simulink model "Automated_BCM_Integrated_2020b"  (R2020b)
settings: Solver=VariableStepAuto  StartTime=0.0  StopTime=100  RelTol=1e-3
undefined symbols (not defined in the file): sigbuilder_block
settings Model: EnablePacing=on  PacingRate=2  Creator=99003729  LastModifiedBy=99003729

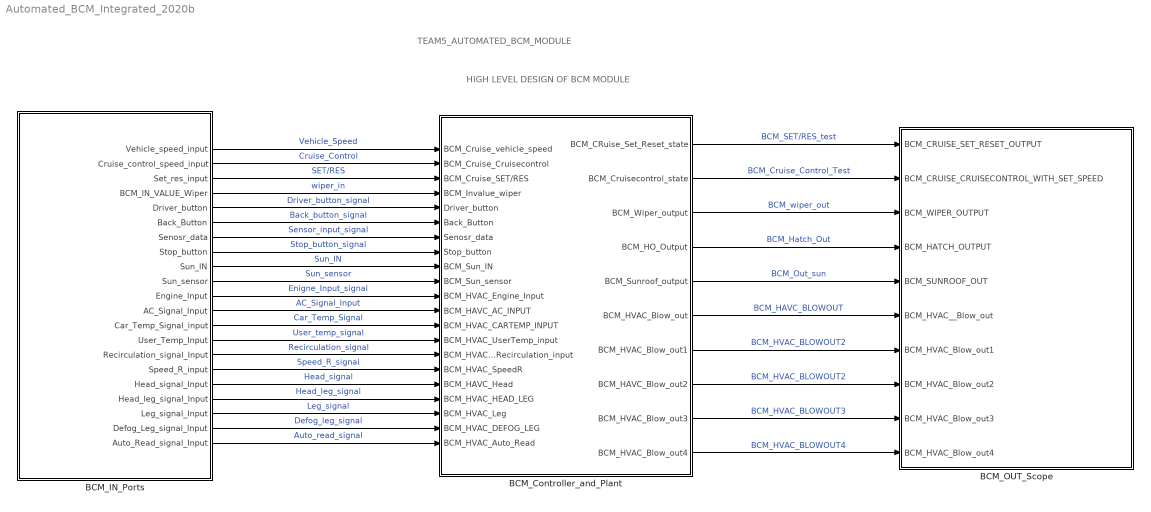
== system Automated_BCM_Integrated_2020b ==
  note: HIGH LEVEL DESIGN OF BCM MODULE
  note: TEAM5_AUTOMATED_BCM_MODULE
  BCM_Controller_and_Plant : Subsystem
  BCM_IN_Ports : Subsystem
  BCM_OUT_Scope : Subsystem
  wires:
  BCM_IN_Ports/1(Vehicle_speed_input) -> BCM_Controller_and_Plant/1(BCM_Cruise_vehicle_speed)  "Vehicle_Speed"
  BCM_IN_Ports/3(Set_res_input) -> BCM_Controller_and_Plant/3(BCM_Cruise_SET/RES)  "SET/RES"
  BCM_IN_Ports/2(Cruise_control_speed_input) -> BCM_Controller_and_Plant/2(BCM_Cruise_Cruisecontrol)  "Cruise_Control"
  BCM_Controller_and_Plant/1(BCM_CRuise_Set_Reset_state) -> BCM_OUT_Scope/1(BCM_CRUISE_SET_RESET_OUTPUT)  "BCM_SET/RES_test"
  BCM_Controller_and_Plant/2(BCM_Cruisecontrol_state) -> BCM_OUT_Scope/2(BCM_CRUISE_CRUISECONTROL_WITH_SET_SPEED)  "BCM_Cruise_Control_Test"
  BCM_IN_Ports/4(BCM_IN_VALUE_Wiper) -> BCM_Controller_and_Plant/4(BCM_Invalue_wiper)  "wiper_in"
  BCM_Controller_and_Plant/3(BCM_Wiper_output) -> BCM_OUT_Scope/3(BCM_WIPER_OUTPUT)  "BCM_wiper_out"
  BCM_Controller_and_Plant/4(BCM_HO_Output) -> BCM_OUT_Scope/4(BCM_HATCH_OUTPUT)  "BCM_Hatch_Out"
  BCM_IN_Ports/5(Driver_button) -> BCM_Controller_and_Plant/5(Driver_button)  "Driver_button_signal"
  BCM_IN_Ports/6(Back_Button) -> BCM_Controller_and_Plant/6(Back_Button)  "Back_button_signal"
  BCM_IN_Ports/7(Senosr_data) -> BCM_Controller_and_Plant/7(Senosr_data)  "Sensor_input_signal"
  BCM_IN_Ports/8(Stop_button) -> BCM_Controller_and_Plant/8(Stop_button)  "Stop_button_signal"
  BCM_Controller_and_Plant/5(BCM_Sunroof_output) -> BCM_OUT_Scope/5(BCM_SUNROOF_OUT)  "BCM_Out_sun"
  BCM_IN_Ports/9(Sun_IN) -> BCM_Controller_and_Plant/9(BCM_Sun_IN)  "Sun_IN"
  BCM_IN_Ports/10(Sun_sensor) -> BCM_Controller_and_Plant/10(BCM_Sun_sensor)  "Sun_sensor"
  BCM_IN_Ports/11(Engine_Input) -> BCM_Controller_and_Plant/11(BCM_HVAC_Engine_Input)  "Enigne_Input_signal"
  BCM_IN_Ports/12(AC_Signal_Input) -> BCM_Controller_and_Plant/12(BCM_HAVC_AC_INPUT)  "AC_Signal_Input"
  BCM_IN_Ports/13(Car_Temp_Signal_input) -> BCM_Controller_and_Plant/13(BCM_HVAC_CARTEMP_INPUT)  "Car_Temp_Signal"
  BCM_IN_Ports/14(User_Temp_Input) -> BCM_Controller_and_Plant/14(BCM_HVAC_UserTemp_input)  "User_temp_signal"
  BCM_IN_Ports/15(Recirculation_signal_Input) -> BCM_Controller_and_Plant/15(BCM_HVAC_Recirculation_input)  "Recirculation_signal"
  BCM_IN_Ports/16(Speed_R_input) -> BCM_Controller_and_Plant/16(BCM_HVAC_SpeedR)  "Speed_R_signal"
  BCM_IN_Ports/17(Head_signal_Input) -> BCM_Controller_and_Plant/17(BCM_HAVC_Head)  "Head_signal"
  BCM_IN_Ports/18(Head_leg_signal_Input) -> BCM_Controller_and_Plant/18(BCM_HVAC_HEAD_LEG)  "Head_leg_signal"
  BCM_IN_Ports/19(Leg_signal_Input) -> BCM_Controller_and_Plant/19(BCM_HVAC_Leg)  "Leg_signal"
  BCM_IN_Ports/20(Defog_Leg_signal_Input) -> BCM_Controller_and_Plant/20(BCM_HVAC_DEFOG_LEG)  "Defog_leg_signal"
  BCM_IN_Ports/21(Auto_Read_signal_Input) -> BCM_Controller_and_Plant/21(BCM_HVAC_Auto_Read)  "Auto_read_signal"
  BCM_Controller_and_Plant/6(BCM_HVAC_Blow_out) -> BCM_OUT_Scope/6(BCM_HVAC__Blow_out)  "BCM_HAVC_BLOWOUT"
  BCM_Controller_and_Plant/7(BCM_HVAC_Blow_out1) -> BCM_OUT_Scope/7(BCM_HVAC_Blow_out1)  "BCM_HVAC_BLOWOUT2"
  BCM_Controller_and_Plant/8(BCM_HAVC_Blow_out2) -> BCM_OUT_Scope/8(BCM_HVAC_Blow_out2)  "BCM_HVAC_BLOWOUT2"
  BCM_Controller_and_Plant/9(BCM_HVAC_Blow_out3) -> BCM_OUT_Scope/9(BCM_HVAC_Blow_out3)  "BCM_HVAC_BLOWOUT3"
  BCM_Controller_and_Plant/10(BCM_HVAC_Blow_out4) -> BCM_OUT_Scope/10(BCM_HVAC_Blow_out4)  "BCM_HVAC_BLOWOUT4"

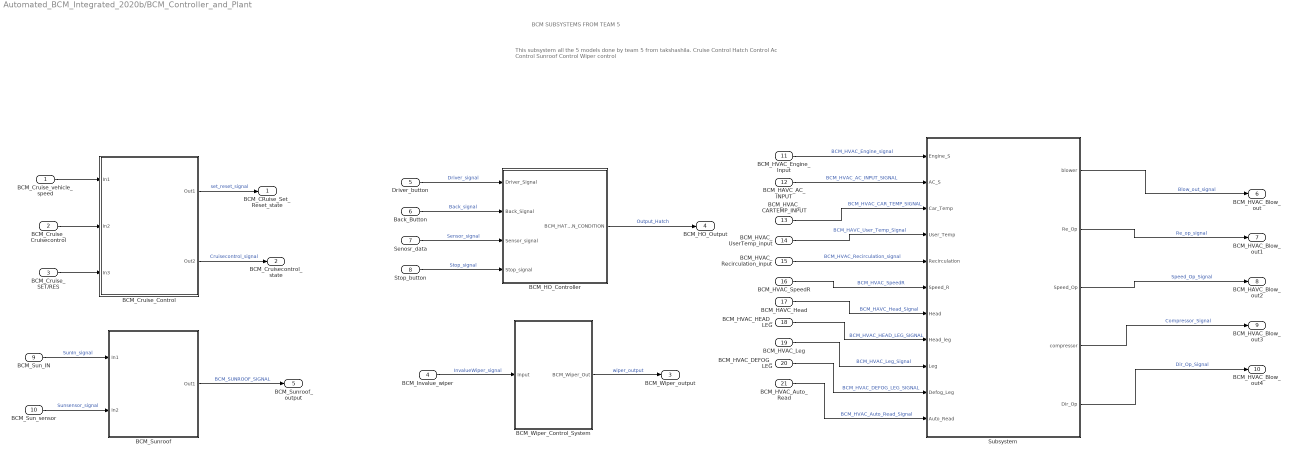
== system Automated_BCM_Integrated_2020b/BCM_Controller_and_Plant ==
  note: This subsystem all the 5 models done by team 5 from takshashila.
      | Cruise Control
      | Hatch Control
      | Ac Control
      | Sunroof Control
      | Wiper control
  note: BCM SUBSYSTEMS FROM TEAM 5
  BCM_Cruise_vehicle_speed : Inport
  BCM_Cruise_Cruisecontrol : Inport  Port=2
  BCM_Cruise_SET/RES : Inport  Port=3
  BCM_Invalue_wiper : Inport  Port=4
  Driver_button : Inport  Port=5
  Back_Button : Inport  Port=6
  Senosr_data : Inport  Port=7
  Stop_button : Inport  Port=8
  BCM_Sun_IN : Inport  Port=9
  BCM_Sun_sensor : Inport  Port=10
  BCM_HVAC_Engine_Input : Inport  Port=11
  BCM_HAVC_AC_INPUT : Inport  Port=12
  BCM_HVAC_CARTEMP_INPUT : Inport  Port=13
  BCM_HVAC_UserTemp_input : Inport  Port=14
  BCM_HVAC_Recirculation_input : Inport  Port=15
  BCM_HVAC_SpeedR : Inport  Port=16
  BCM_HAVC_Head : Inport  Port=17
  BCM_HVAC_HEAD_LEG : Inport  Port=18
  BCM_HVAC_Leg : Inport  Port=19
  BCM_HVAC_DEFOG_LEG : Inport  Port=20
  BCM_HVAC_Auto_Read : Inport  Port=21
  BCM_Cruise_Control : Subsystem
  BCM_HO_Controller : Subsystem
  BCM_Sunroof : Subsystem
  BCM_Wiper_Control_System : Subsystem
  Subsystem : Subsystem
  BCM_CRuise_Set_Reset_state : Outport
  BCM_Cruisecontrol_state : Outport  Port=2
  BCM_Wiper_output : Outport  Port=3
  BCM_HO_Output : Outport  Port=4
  BCM_Sunroof_output : Outport  Port=5
  BCM_HVAC_Blow_out : Outport  Port=6
  BCM_HVAC_Blow_out1 : Outport  Port=7
  BCM_HAVC_Blow_out2 : Outport  Port=8
  BCM_HVAC_Blow_out3 : Outport  Port=9
  BCM_HVAC_Blow_out4 : Outport  Port=10
  wires:
  BCM_Cruise_vehicle_speed/1 -> BCM_Cruise_Control/1(In1)
  BCM_Cruise_Cruisecontrol/1 -> BCM_Cruise_Control/2(In2)
  BCM_Cruise_SET/RES/1 -> BCM_Cruise_Control/3(In3)
  BCM_Cruise_Control/1(Out1) -> BCM_CRuise_Set_Reset_state/1  "set_reset_signal"
  BCM_Cruise_Control/2(Out2) -> BCM_Cruisecontrol_state/1  "Cruisecontrol_signal"
  Driver_button/1 -> BCM_HO_Controller/1(Driver_Signal)  "Driver_signal"
  Back_Button/1 -> BCM_HO_Controller/2(Back_Signal)  "Back_signal"
  Senosr_data/1 -> BCM_HO_Controller/3(Sensor_signal)  "Sensor_signal"
  Stop_button/1 -> BCM_HO_Controller/4(Stop_signal)  "Stop_signal"
  BCM_Sunroof/1(Out1) -> BCM_Sunroof_output/1  "BCM_SUNROOF_SIGNAL"
  BCM_Sun_IN/1 -> BCM_Sunroof/1(In1)  "SunIn_signal"
  BCM_Sun_sensor/1 -> BCM_Sunroof/2(In2)  "Sunsensor_signal"
  BCM_Invalue_wiper/1 -> BCM_Wiper_Control_System/1(Input)  "InvalueWiper_signal"
  BCM_Wiper_Control_System/1(BCM_Wiper_Out) -> BCM_Wiper_output/1  "wiper_output"
  BCM_HO_Controller/1(BCM_HATCHOPEN_CONDITION) -> BCM_HO_Output/1  "Output_Hatch"
  BCM_HVAC_Engine_Input/1 -> Subsystem/1(Engine_S)  "BCM_HVAC_Engine_signal"
  BCM_HAVC_AC_INPUT/1 -> Subsystem/2(AC_S)  "BCM_HVAC_AC_INPUT_SIGNAL"
  BCM_HVAC_CARTEMP_INPUT/1 -> Subsystem/3(Car_Temp)  "BCM_HVAC_CAR_TEMP_SIGNAL"
  BCM_HVAC_UserTemp_input/1 -> Subsystem/4(User_Temp)  "BCM_HAVC_User_Temp_Signal"
  BCM_HVAC_Recirculation_input/1 -> Subsystem/5(Recirculation)  "BCM_HVAC_Recirculation_signal"
  BCM_HVAC_SpeedR/1 -> Subsystem/6(Speed_R)  "BCM_HVAC_SpeedR"
  BCM_HAVC_Head/1 -> Subsystem/7(Head)  "BCM_HAVC_Head_Signal"
  BCM_HVAC_HEAD_LEG/1 -> Subsystem/8(Head_leg)  "BCM_HVAC_HEAD_LEG_SIGNAL"
  BCM_HVAC_Leg/1 -> Subsystem/9(Leg)  "BCM_HVAC_Leg_Signal"
  BCM_HVAC_DEFOG_LEG/1 -> Subsystem/10(Defog_Leg)  "BCM_HVAC_DEFOG_LEG_SIGNAL"
  BCM_HVAC_Auto_Read/1 -> Subsystem/11(Auto_Read)  "BCM_HVAC_Auto_Read_Signal"
  Subsystem/1(blower) -> BCM_HVAC_Blow_out/1  "Blow_out_signal"
  Subsystem/2(Re_Op) -> BCM_HVAC_Blow_out1/1  "Re_op_signal"
  Subsystem/3(Speed_Op) -> BCM_HAVC_Blow_out2/1  "Speed_Op_Signal"
  Subsystem/4(compressor) -> BCM_HVAC_Blow_out3/1  "Compressor_Signal"
  Subsystem/5(Dir_Op) -> BCM_HVAC_Blow_out4/1  "Dir_Op_Signal"

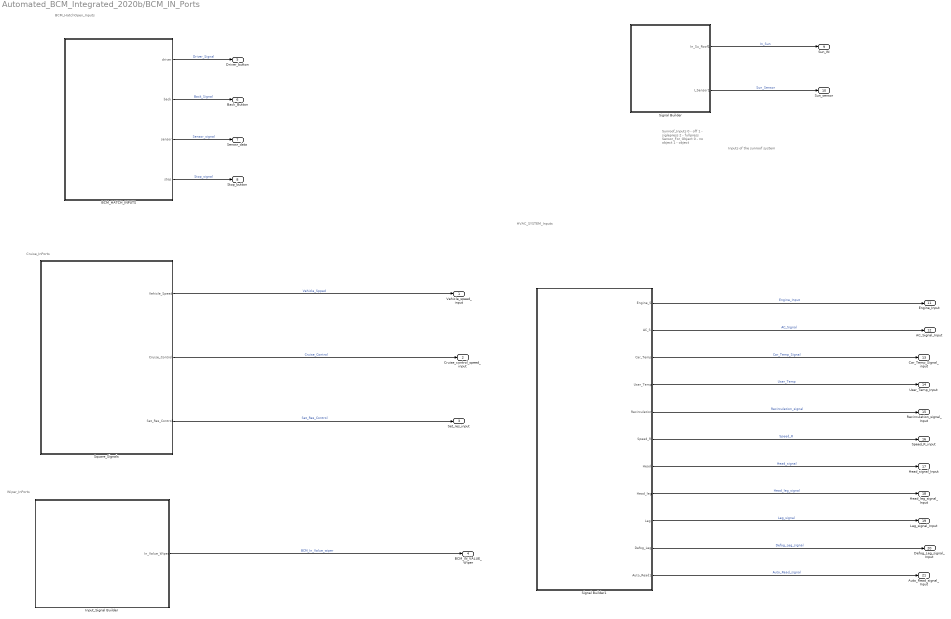
== system Automated_BCM_Integrated_2020b/BCM_IN_Ports ==
  note: HVAC_SYSTEM_Inputs
  note: BCM_HatchOpen_Inputs
  note: Wiper_InPorts
  note: Cruise_InPorts
  note: Inputs of the sunroof system
  note: Sunroof_Inputs
      | 0 - off
      | 1 - siglepress
      | 2 - fullpress
      | Sensor_For_Object
      | 0 - no object
      | 1 - object
  BCM_HATCH_INPUTS : Subsystem  Tag=STV Subsys  LoadFcn=sigbuilder_block('load');  StartFcn=sigbuilder_block('start');  StopFcn=sigbuilder_block('stop');  ClipboardFcn=sigbuilder_block('clipboard');  mask(Sigbuilder block){tuvar=[0:10]}
      mask help: Simulink:masks:SigbuilderBlock_MD
      mask init:
      | if ~strcmp(get_param(bdroot(gcbh),'SimulationStatus'),'stopped') tuvar = sigbuilder_block('maskInit'); end
      settings: CopyFcn=sigbuilder_block('copy');  DeleteFcn=sigbuilder_block('delete');  ModelCloseFcn=sigbuilder_block('modelClose');  PreSaveFcn=sigbuilder_block('preSave');  PauseFcn=sigbuilder_block('pause');  ContinueFcn=sigbuilder_block('continue');  NameChangeFcn=sigbuilder_block('namechange');  OpenFcn=sigbuilder_block('open',[0 30 1440 722.25 ]);  CloseFcn=sigbuilder_block('close');
      mask Display: plot(0, 0, 100, 100,[2, 2, 32, 32, 2], [68, 8, 8, 68, 68],[32, 2], [38, 38], [32, 19, 2],[53, 60, 44], [32, 17, 17, 2],[16, 16, 31, 31]);txt = getActiveGroup(gcbh);text(2, 100, txt,'verticalAlignment', 'top');
  Input_Signal Builder : Subsystem  Tag=STV Subsys  LoadFcn=sigbuilder_block('load');  StartFcn=sigbuilder_block('start');  StopFcn=sigbuilder_block('stop');  ClipboardFcn=sigbuilder_block('clipboard');  mask(Sigbuilder block){tuvar=[0:10]}
      mask help: Simulink:masks:SigbuilderBlock_MD
      mask init:
      | if ~strcmp(get_param(bdroot(gcbh),'SimulationStatus'),'stopped') tuvar = sigbuilder_block('maskInit'); end
      settings: CopyFcn=sigbuilder_block('copy');  DeleteFcn=sigbuilder_block('delete');  ModelCloseFcn=sigbuilder_block('modelClose');  PreSaveFcn=sigbuilder_block('preSave');  PauseFcn=sigbuilder_block('pause');  ContinueFcn=sigbuilder_block('continue');  NameChangeFcn=sigbuilder_block('namechange');  OpenFcn=sigbuilder_block('open',[339 188.25 550.5 359.25 ]);  CloseFcn=sigbuilder_block('close');
      mask Display: plot(0, 0, 100, 100,[2, 2, 32, 32, 2], [68, 8, 8, 68, 68],[32, 2], [38, 38], [32, 19, 2],[53, 60, 44], [32, 17, 17, 2],[16, 16, 31, 31]);txt = getActiveGroup(gcbh);text(2, 100, txt,'verticalAlignment', 'top');
  Signal Builder : Subsystem  Tag=STV Subsys  LoadFcn=sigbuilder_block('load');  StartFcn=sigbuilder_block('start');  StopFcn=sigbuilder_block('stop');  ClipboardFcn=sigbuilder_block('clipboard');  mask(Sigbuilder block){tuvar=[0:10]}
      mask help: Simulink:masks:SigbuilderBlock_MD
      mask init:
      | if ~strcmp(get_param(bdroot(gcbh),'SimulationStatus'),'stopped') tuvar = sigbuilder_block('maskInit'); end
      settings: CopyFcn=sigbuilder_block('copy');  DeleteFcn=sigbuilder_block('delete');  ModelCloseFcn=sigbuilder_block('modelClose');  PreSaveFcn=sigbuilder_block('preSave');  PauseFcn=sigbuilder_block('pause');  ContinueFcn=sigbuilder_block('continue');  NameChangeFcn=sigbuilder_block('namechange');  OpenFcn=sigbuilder_block('open',[534 -108 550.5 359.25 ]);  CloseFcn=sigbuilder_block('close');
      mask Display: plot(0, 0, 100, 100,[2, 2, 32, 32, 2], [68, 8, 8, 68, 68],[32, 2], [38, 38], [32, 19, 2],[53, 60, 44], [32, 17, 17, 2],[16, 16, 31, 31]);txt = getActiveGroup(gcbh);text(2, 100, txt,'verticalAlignment', 'top');
  Signal Builder1 : Subsystem  Tag=STV Subsys  LoadFcn=sigbuilder_block('load');  StartFcn=sigbuilder_block('start');  StopFcn=sigbuilder_block('stop');  ClipboardFcn=sigbuilder_block('clipboard');  mask(Sigbuilder block){tuvar=[0:10]}
      mask help: Simulink:masks:SigbuilderBlock_MD
      mask init:
      | if ~strcmp(get_param(bdroot(gcbh),'SimulationStatus'),'stopped') tuvar = sigbuilder_block('maskInit'); end
      settings: CopyFcn=sigbuilder_block('copy');  DeleteFcn=sigbuilder_block('delete');  ModelCloseFcn=sigbuilder_block('modelClose');  PreSaveFcn=sigbuilder_block('preSave');  PauseFcn=sigbuilder_block('pause');  ContinueFcn=sigbuilder_block('continue');  NameChangeFcn=sigbuilder_block('namechange');  OpenFcn=sigbuilder_block('open',[417 237.75 550.5 399.75 ]);  CloseFcn=sigbuilder_block('close');
      mask Display: plot(0, 0, 100, 100,[2, 2, 32, 32, 2], [68, 8, 8, 68, 68],[32, 2], [38, 38], [32, 19, 2],[53, 60, 44], [32, 17, 17, 2],[16, 16, 31, 31]);txt = getActiveGroup(gcbh);text(2, 100, txt,'verticalAlignment', 'top');
  Square_Signals : Subsystem  Tag=STV Subsys  LoadFcn=sigbuilder_block('load');  StartFcn=sigbuilder_block('start');  StopFcn=sigbuilder_block('stop');  ClipboardFcn=sigbuilder_block('clipboard');  mask(Sigbuilder block){tuvar=[0:10]}
      mask help: Simulink:masks:SigbuilderBlock_MD
      mask init:
      | if ~strcmp(get_param(bdroot(gcbh),'SimulationStatus'),'stopped') tuvar = sigbuilder_block('maskInit'); end
      settings: CopyFcn=sigbuilder_block('copy');  DeleteFcn=sigbuilder_block('delete');  ModelCloseFcn=sigbuilder_block('modelClose');  PreSaveFcn=sigbuilder_block('preSave');  PauseFcn=sigbuilder_block('pause');  ContinueFcn=sigbuilder_block('continue');  NameChangeFcn=sigbuilder_block('namechange');  OpenFcn=sigbuilder_block('open',[0.75 30.75 718.5 715.5 ]);  CloseFcn=sigbuilder_block('close');
      mask Display: plot(0, 0, 100, 100,[2, 2, 32, 32, 2], [68, 8, 8, 68, 68],[32, 2], [38, 38], [32, 19, 2],[53, 60, 44], [32, 17, 17, 2],[16, 16, 31, 31]);txt = getActiveGroup(gcbh);text(2, 100, txt,'verticalAlignment', 'top');
  Vehicle_speed_input : Outport
  Cruise_control_speed_input : Outport  Port=2
  Set_res_input : Outport  Port=3
  BCM_IN_VALUE_Wiper : Outport  Port=4
  Driver_button : Outport  Port=5
  Back_Button : Outport  Port=6
  Senosr_data : Outport  Port=7
  Stop_button : Outport  Port=8
  Sun_IN : Outport  Port=9
  Sun_sensor : Outport  Port=10
  Engine_Input : Outport  Port=11
  AC_Signal_Input : Outport  Port=12
  Car_Temp_Signal_input : Outport  Port=13
  User_Temp_Input : Outport  Port=14
  Recirculation_signal_Input : Outport  Port=15
  Speed_R_input : Outport  Port=16
  Head_signal_Input : Outport  Port=17
  Head_leg_signal_Input : Outport  Port=18
  Leg_signal_Input : Outport  Port=19
  Defog_Leg_signal_Input : Outport  Port=20
  Auto_Read_signal_Input : Outport  Port=21
  wires:
  Square_Signals/2(Cruise_Control) -> Cruise_control_speed_input/1  "Cruise_Control"
  Square_Signals/1(Vehicle_Speed) -> Vehicle_speed_input/1  "Vehicle_Spped"
  Square_Signals/3(Set_Res_Control) -> Set_res_input/1  "Set_Res_Control"
  Input_Signal Builder/1(In_Value_Wiper) -> BCM_IN_VALUE_Wiper/1  "BCM_In_Value_wiper"
  BCM_HATCH_INPUTS/4(stop) -> Stop_button/1  "Stop_signal"
  BCM_HATCH_INPUTS/3(sensor) -> Senosr_data/1  "Sensor_signal"
  BCM_HATCH_INPUTS/2(back) -> Back_Button/1  "Back_Signal"
  BCM_HATCH_INPUTS/1(driver) -> Driver_button/1  "Driver_Signal"
  Signal Builder/1(In_Su_Roof1) -> Sun_IN/1  "In_Sun"
  Signal Builder/2(I_Sensor1) -> Sun_sensor/1  "Sun_Sensor"
  Signal Builder1/8(Head_leg) -> Head_leg_signal_Input/1  "Head_leg_signal"
  Signal Builder1/9(Leg) -> Leg_signal_Input/1  "Leg_signal"
  Signal Builder1/4(User_Temp) -> User_Temp_Input/1  "User_Temp"
  Signal Builder1/6(Speed_R) -> Speed_R_input/1  "Speed_R"
  Signal Builder1/7(Head) -> Head_signal_Input/1  "Head_signal"
  Signal Builder1/3(Car_Temp) -> Car_Temp_Signal_input/1  "Car_Temp_Signal"
  Signal Builder1/10(Defog_Leg) -> Defog_Leg_signal_Input/1  "Defog_Leg_signal"
  Signal Builder1/5(Recirculation) -> Recirculation_signal_Input/1  "Recirculation_signal"
  Signal Builder1/11(Auto_Read1) -> Auto_Read_signal_Input/1  "Auto_Read_signal"
  Signal Builder1/2(AC_S) -> AC_Signal_Input/1  "AC_Signal"
  Signal Builder1/1("      Engine_S  ") -> Engine_Input/1  "Engine_Input"

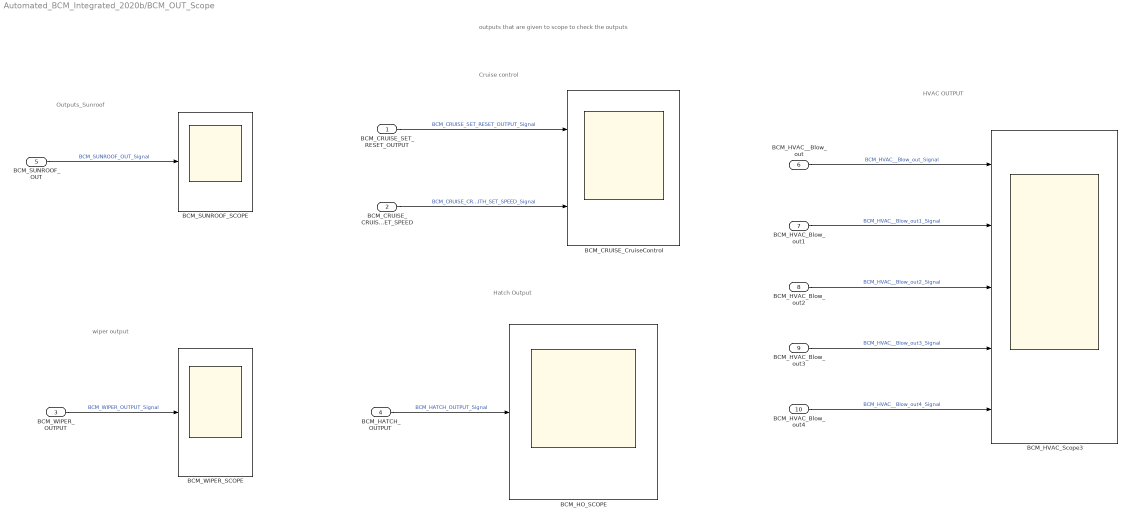
== system Automated_BCM_Integrated_2020b/BCM_OUT_Scope ==
  note: HVAC OUTPUT
  note: wiper output
  note: Hatch Output
  note: Cruise control
  note: Outputs_Sunroof
  note: outputs that are given to scope to check the outputs
  BCM_CRUISE_SET_RESET_OUTPUT : Inport
  BCM_CRUISE_CRUISECONTROL_WITH_SET_SPEED : Inport  Port=2
  BCM_WIPER_OUTPUT : Inport  Port=3
  BCM_HATCH_OUTPUT : Inport  Port=4
  BCM_SUNROOF_OUT : Inport  Port=5
  BCM_HVAC__Blow_out : Inport  Port=6
  BCM_HVAC_Blow_out1 : Inport  Port=7
  BCM_HVAC_Blow_out2 : Inport  Port=8
  BCM_HVAC_Blow_out3 : Inport  Port=9
  BCM_HVAC_Blow_out4 : Inport  Port=10
  BCM_CRUISE_CruiseControl : Scope  NumInputPorts=2
  BCM_HO_SCOPE : Scope
  BCM_HVAC_Scope3 : Scope  NumInputPorts=5
  BCM_SUNROOF_SCOPE : Scope
  BCM_WIPER_SCOPE : Scope
  wires:
  BCM_WIPER_OUTPUT/1 -> BCM_WIPER_SCOPE/1  "BCM_WIPER_OUTPUT_Signal"
  BCM_SUNROOF_OUT/1 -> BCM_SUNROOF_SCOPE/1  "BCM_SUNROOF_OUT_Signal"
  BCM_CRUISE_SET_RESET_OUTPUT/1 -> BCM_CRUISE_CruiseControl/1  "BCM_CRUISE_SET_RESET_OUTPUT_Signal"
  BCM_CRUISE_CRUISECONTROL_WITH_SET_SPEED/1 -> BCM_CRUISE_CruiseControl/2  "BCM_CRUISE_CRUISECONTROL_WITH_SET_SPEED_Signal"
  BCM_HATCH_OUTPUT/1 -> BCM_HO_SCOPE/1  "BCM_HATCH_OUTPUT_Signal"
  BCM_HVAC_Blow_out4/1 -> BCM_HVAC_Scope3/5  "BCM_HVAC__Blow_out4_Signal"
  BCM_HVAC_Blow_out2/1 -> BCM_HVAC_Scope3/3  "BCM_HVAC__Blow_out2_Signal"
  BCM_HVAC__Blow_out/1 -> BCM_HVAC_Scope3/1  "BCM_HVAC__Blow_out_Signal"
  BCM_HVAC_Blow_out3/1 -> BCM_HVAC_Scope3/4  "BCM_HVAC__Blow_out3_Signal"
  BCM_HVAC_Blow_out1/1 -> BCM_HVAC_Scope3/2  "BCM_HVAC__Blow_out1_Signal"

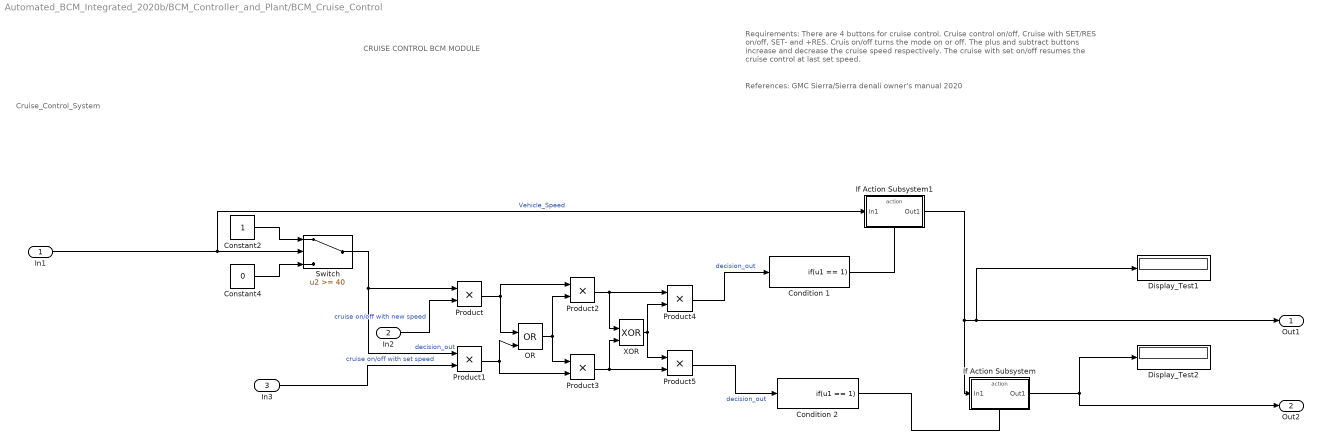
== system Automated_BCM_Integrated_2020b/BCM_Controller_and_Plant/BCM_Cruise_Control ==
  note: Cruise_Control_System
  note: CRUISE CONTROL BCM MODULE
  note: References: GMC Sierra/Sierra denali owner's manual 2020
  note: Requirements: There are 4 buttons for cruise control. Cruise control on/off, Cruise with SET/RES on/off, SET- and +RES. Cruis on/off turns the mode on or off. The plus and subtract buttons increase and decrease the cruise speed respectively. The cruise with set on/off resumes the cruise control at last set speed.
  In1 : Inport
  In2 : Inport  Port=2
  In3 : Inport  Port=3
  Condition 1 : If  IfExpression=u1 == 1  ShowElse=off
  Condition 2 : If  IfExpression=u1 == 1  ShowElse=off
  Constant2 : Constant
  Constant4 : Constant  Value=0
  Display_Test1 : Display
  Display_Test2 : Display
  If Action Subsystem : Subsystem  TreatAsAtomicUnit=on
  If Action Subsystem1 : Subsystem  TreatAsAtomicUnit=on
  OR : Logic  Operator=OR  IconShape=distinctive  AllPortsSameDT=off  OutDataTypeStr=boolean
  Product{,1..5} (6 alike) : Product
  Switch : Switch  Threshold=40
  XOR : Logic  Operator=XOR  IconShape=distinctive  AllPortsSameDT=off  OutDataTypeStr=boolean
  Out1 : Outport
  Out2 : Outport  Port=2
  wires:
  In3/1 -> Product1/2  "cruise on/off with set speed"
  Product5/1 -> Condition 2/1  "decision_out"
  Condition 1/1 -> If Action Subsystem1/Action
  Condition 2/1 -> If Action Subsystem/Action
  If Action Subsystem/1(Out1) -> Display_Test2/1, Out2/1
  Product2/1 -> Product4/1, XOR/1
  XOR/1 -> Product4/2, Product5/1
  In1/1 -> Switch/2, If Action Subsystem1/1(In1)  "Vehicle_Speed"
  OR/1 -> Product3/1, Product2/2
  Product/1 -> Product2/1, OR/1
  In2/1 -> Product/2  "cruise on/off with new speed"
  Constant4/1 -> Switch/3
  Product1/1 -> OR/2, Product3/2
  Product3/1 -> Product5/2, XOR/2
  Switch/1 -> Product1/1, Product/1  "decision_out"
  Constant2/1 -> Switch/1
  Product4/1 -> Condition 1/1  "decision_out"
  If Action Subsystem1/1(Out1) -> If Action Subsystem/1(In1), Out1/1, Display_Test1/1

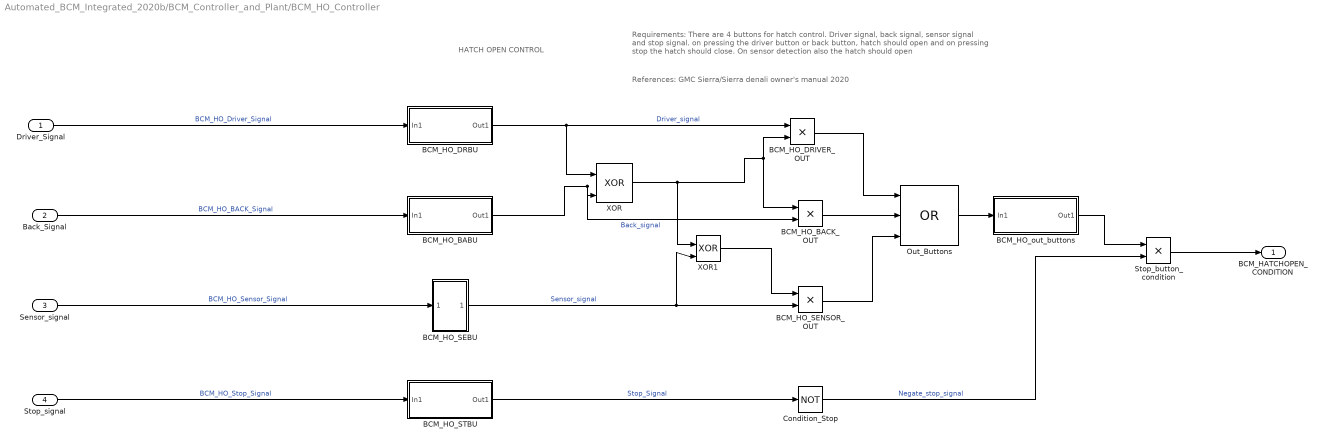
== system Automated_BCM_Integrated_2020b/BCM_Controller_and_Plant/BCM_HO_Controller ==
  note: HATCH OPEN CONTROL
  note: References: GMC Sierra/Sierra denali owner's manual 2020
  note: Requirements: There are 4 buttons for hatch control. Driver signal, back signal, sensor signal and stop signal. on pressing the driver button or back button, hatch should open and on pressing stop the hatch should close. On sensor detection also the hatch should open
  Driver_Signal : Inport
  Back_Signal : Inport  Port=2
  Sensor_signal : Inport  Port=3
  Stop_signal : Inport  Port=4
  BCM_HO_BABU : Subsystem
  BCM_HO_BACK_OUT : Product
  BCM_HO_DRBU : Subsystem
  BCM_HO_DRIVER_OUT : Product
  BCM_HO_SEBU : Subsystem
  BCM_HO_SENSOR_OUT : Product
  BCM_HO_STBU : Subsystem
  BCM_HO_out_buttons : Subsystem
  Condition_Stop : Logic  Operator=NOT  IconShape=distinctive  AllPortsSameDT=off  OutDataTypeStr=boolean
  Out_Buttons : Logic  Operator=OR  Inputs=3  IconShape=distinctive  AllPortsSameDT=off  OutDataTypeStr=boolean
  Stop_button_condition : Product
  XOR : Logic  Operator=XOR  IconShape=distinctive  AllPortsSameDT=off  OutDataTypeStr=boolean
  XOR1 : Logic  Operator=XOR  IconShape=distinctive  AllPortsSameDT=off  OutDataTypeStr=boolean
  BCM_HATCHOPEN_CONDITION : Outport
  wires:
  BCM_HO_SEBU/1(Out1) -> BCM_HO_SENSOR_OUT/2, XOR1/2  "Sensor_signal"
  Stop_signal/1 -> BCM_HO_STBU/1(In1)  "BCM_HO_Stop_Signal"
  XOR/1 -> XOR1/1, BCM_HO_BACK_OUT/1, BCM_HO_DRIVER_OUT/2
  XOR1/1 -> BCM_HO_SENSOR_OUT/1
  BCM_HO_BABU/1(Out1) -> BCM_HO_BACK_OUT/2, XOR/2  "Back_signal"
  Out_Buttons/1 -> BCM_HO_out_buttons/1(In1)
  BCM_HO_STBU/1(Out1) -> Condition_Stop/1  "Stop_Signal"
  BCM_HO_out_buttons/1(Out1) -> Stop_button_condition/1
  BCM_HO_DRBU/1(Out1) -> BCM_HO_DRIVER_OUT/1, XOR/1  "Driver_signal"
  Sensor_signal/1 -> BCM_HO_SEBU/1(In1)  "BCM_HO_Sensor_Signal"
  Driver_Signal/1 -> BCM_HO_DRBU/1(In1)  "BCM_HO_Driver_Signal"
  Back_Signal/1 -> BCM_HO_BABU/1(In1)  "BCM_HO_BACK_Signal"
  BCM_HO_DRIVER_OUT/1 -> Out_Buttons/1
  Condition_Stop/1 -> Stop_button_condition/2  "Negate_stop_signal"
  Stop_button_condition/1 -> BCM_HATCHOPEN_CONDITION/1
  BCM_HO_SENSOR_OUT/1 -> Out_Buttons/3
  BCM_HO_BACK_OUT/1 -> Out_Buttons/2

== system Automated_BCM_Integrated_2020b/BCM_Controller_and_Plant/BCM_Sunroof ==
  note: Requirements:
      | 1)Sunroof open/close: Press push buttons open or close.
      | 2)Open: If open push button is pressed sunroof open.
      | 3)Close: If close push button is pressed sunroof close.
  note: SUNROOF CONTROL BCM MODULE
  note: References: GMC Sierra/Sierra denali owner's manual 2020
  In1 : Inport
  In2 : Inport  Port=2
  Function_Sun : MATLAB Function  TreatAsAtomicUnit=on
  Out1 : Outport
  wires:
  Function_Sun/1(y) -> Out1/1  "BCM_Out_Sun"
  In2/1 -> Function_Sun/2(v)  "BCM_Sun_Sensor"
  In1/1 -> Function_Sun/1(u)  "BCM_Sun_In"

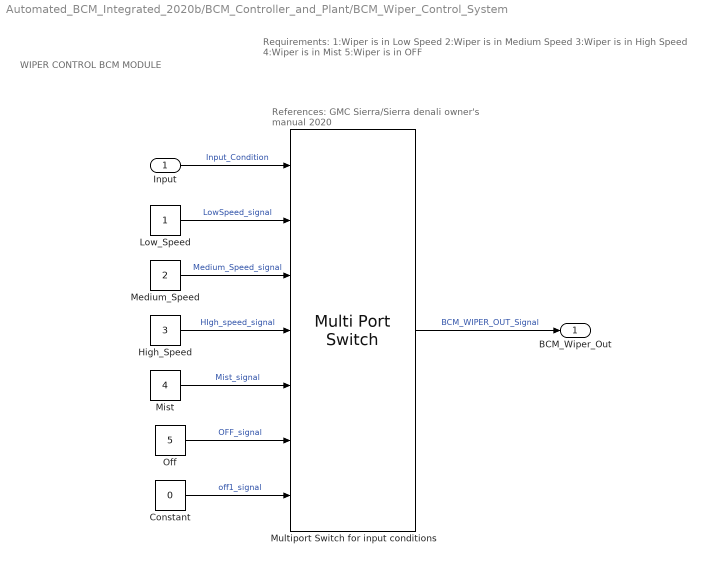
== system Automated_BCM_Integrated_2020b/BCM_Controller_and_Plant/BCM_Wiper_Control_System ==
  note: References: GMC Sierra/Sierra denali owner's manual 2020
  note: WIPER CONTROL BCM MODULE
  note: Requirements:
      | 1:Wiper is in Low Speed
      | 2:Wiper is in Medium Speed
      | 3:Wiper is in High Speed
      | 4:Wiper is in Mist
      | 5:Wiper is in OFF
  Input : Inport
  Constant : Constant  Value=0
  High_Speed : Constant  Value=3
  Low_Speed : Constant
  Medium_Speed : Constant  Value=2
  Mist : Constant  Value=4
  Multiport Switch for input conditions : MultiPortSwitch  Inputs=6  DiagnosticForDefault=None
  Off : Constant  Value=5
  BCM_Wiper_Out : Outport
  wires:
  Input/1 -> Multiport Switch for input conditions/1  "Input_Condition"
  Low_Speed/1 -> Multiport Switch for input conditions/2  "LowSpeed_signal"
  Mist/1 -> Multiport Switch for input conditions/5  "Mist_signal"
  Medium_Speed/1 -> Multiport Switch for input conditions/3  "Medium_Speed_signal"
  Multiport Switch for input conditions/1 -> BCM_Wiper_Out/1  "BCM_WIPER_OUT_Signal"
  High_Speed/1 -> Multiport Switch for input conditions/4  "HIgh_speed_signal"
  Off/1 -> Multiport Switch for input conditions/6  "OFF_signal"
  Constant/1 -> Multiport Switch for input conditions/7  "off1_signal"

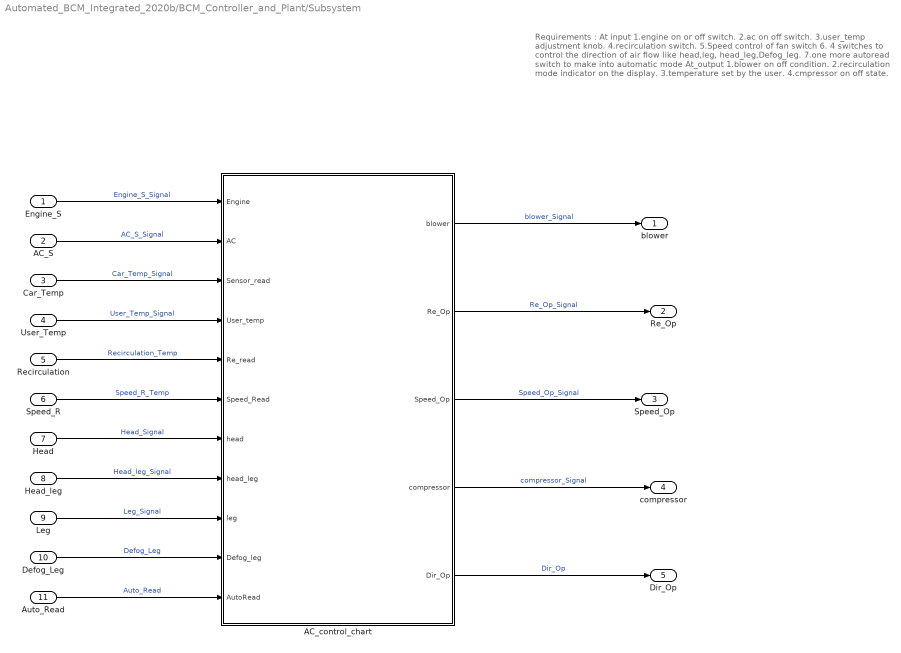
== system Automated_BCM_Integrated_2020b/BCM_Controller_and_Plant/Subsystem ==
  note: Requirements :
      | At input
      | 1.engine on or off switch.
      | 2.ac on off switch.
      | 3.user_temp adjustment knob.
      | 4.recirculation switch.
      | 5.Speed control of fan switch
      | 6. 4 switches to control the direction of air flow like head,leg, head_leg,Defog_leg.
      | 7.one more autoread switch to make into automatic mode
      | At_output
      | 1.blower on off condition.
      | 2.recirculation mode indicator on the display.
      | 3.temperature set by the user.
      | 4.cmpressor on off state.
  Engine_S : Inport
  AC_S : Inport  Port=2
  Car_Temp : Inport  Port=3
  User_Temp : Inport  Port=4
  Recirculation : Inport  Port=5
  Speed_R : Inport  Port=6
  Head : Inport  Port=7
  Head_leg : Inport  Port=8
  Leg : Inport  Port=9
  Defog_Leg : Inport  Port=10
  Auto_Read : Inport  Port=11
  AC_control_chart : Stateflow chart  TreatAsAtomicUnit=on
  blower : Outport
  Re_Op : Outport  Port=2
  Speed_Op : Outport  Port=3
  compressor : Outport  Port=4
  Dir_Op : Outport  Port=5
  wires:
  AC_control_chart/5(Dir_Op) -> Dir_Op/1  "Dir_Op"
  Speed_R/1 -> AC_control_chart/6(Speed_Read)  "Speed_R_Temp"
  Car_Temp/1 -> AC_control_chart/3(Sensor_read)  "Car_Temp_Signal"
  AC_control_chart/4(compressor) -> compressor/1  "compressor_Signal"
  Engine_S/1 -> AC_control_chart/1(Engine)  "Engine_S_Signal"
  Defog_Leg/1 -> AC_control_chart/10(Defog_leg)  "Defog_Leg"
  Head/1 -> AC_control_chart/7(head)  "Head_Signal"
  Head_leg/1 -> AC_control_chart/8(head_leg)  "Head_leg_Signal"
  Leg/1 -> AC_control_chart/9(leg)  "Leg_Signal"
  Recirculation/1 -> AC_control_chart/5(Re_read)  "Recirculation_Temp"
  AC_control_chart/3(Speed_Op) -> Speed_Op/1  "Speed_Op_Signal"
  AC_control_chart/1(blower) -> blower/1  "blower_Signal"
  AC_S/1 -> AC_control_chart/2(AC)  "AC_S_Signal"
  Auto_Read/1 -> AC_control_chart/11(AutoRead)  "Auto_Read"
  User_Temp/1 -> AC_control_chart/4(User_temp)  "User_Temp_Signal"
  AC_control_chart/2(Re_Op) -> Re_Op/1  "Re_Op_Signal"

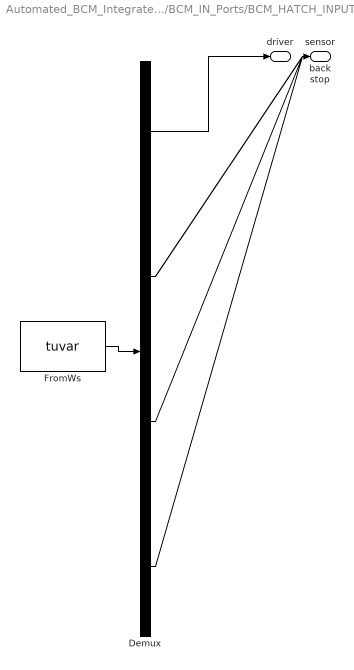
== system Automated_BCM_Integrated_2020b/BCM_IN_Ports/BCM_HATCH_INPUTS ==
  Demux : Demux  Tag=STV Demux
      settings: DisplayOption=none
  FromWs : FromWorkspace  Tag=STV FromWs  VariableName=tuvar
      SigBuilderData=|
      | common.afterFinalStr = 'Extrapolate'
      | common.sampleTime = 0
      | dataSet.timeRange = [0 10]
      | dataSet.name = 'Group 1'
      | sbobj.Groups.Name = 'Group 1'
      | sbobj.Groups.Signals(1).Name = 'driver'
      | sbobj.Groups.Signals(1).XData = [0 5 10 15 20 20 25 30 35 40 40 45 50 55 60 60 65 70 75 80 80 85 90 95 100]
      | sbobj.Groups.Signals(1).YData = [0 0 0 0 0 1 1 1 1 1 0 0 0 0 0 1 1 1 1 1 0 0 0 0 0]
      | sbobj.Groups.Signals(2).Name = 'back'
      | sbobj.Groups.Signals(2).XData = [0 5 10 10 15 20 20 25 30 30 35 40 40 45 50 50 55 60 60 65 70 70 75 80 80 85 90 90 95 100]
      | sbobj.Groups.Signals(2).YData = [0 0 0 1 1 1 0 0 0 1 1 1 0 0 0 1 1 1 0 0 0 1 1 1 0 0 0 1 1 1]
      | sbobj.Groups.Signals(3).Name = 'sensor'
      | sbobj.Groups.Signals(3).XData = [0 5 5 10 10 15 20 20 25 30 35 35 40 40 45 45 50 50 55 55 60 60 65 65 70 70 75 75 80 80 85 85 90 90 95 95 100]
      | sbobj.Groups.Signals(3).YData = [0.9 2.1 3.6 2.31 2 2.1 2.1 0 0 0 2.1 3.6 6.2 2.6 2.3 1.9 0.7 2.3 2.1 3.6 3.8 2.6 2.95 2.3 1.9 3.9 4.9 2 2.1 0.9 1.8 3.756 4.56 1.8 1.96 2.85 2.986]
      | sbobj.Groups.Signals(4).Name = 'stop'
      | sbobj.Groups.Signals(4).XData = [0 5 10 10 15 15 20 20 25 25 30 30 35 35 40 40 45 45 50 50 55 55 60 60 65 65 70 70 75 75 80 80 85 85 90 90 95 95 100]
      | sbobj.Groups.Signals(4).YData = [0 0 1 0 1 0 1 0 1 0 1 0 1 0 1 0 1 0 1 0 1 0 1 0 1 0 1 0 1 0 1 0 1 0 1 0 1 0 1]
      | sbobj.Groups.TimeRange = [0 100]
  driver : Outport  Tag=STV Outport
  back : Outport  Tag=STV Outport  Port=2
  sensor : Outport  Tag=STV Outport  Port=3
  stop : Outport  Tag=STV Outport  Port=4
  wires:
  FromWs/1 -> Demux/1
  Demux/1 -> driver/1
  Demux/2 -> back/1
  Demux/3 -> sensor/1
  Demux/4 -> stop/1

== system Automated_BCM_Integrated_2020b/BCM_IN_Ports/Input_Signal Builder ==
  Demux : Demux  Tag=STV Demux  Outputs=1
      settings: DisplayOption=none
  FromWs : FromWorkspace  Tag=STV FromWs  VariableName=tuvar
      SigBuilderData=|
      | common.afterFinalStr = 'Extrapolate'
      | common.sampleTime = 0
      | dataSet.timeRange = [0 25]
      | dataSet.name = 'Group 1'
      | sbobj.Groups.Name = 'Group 1'
      | sbobj.Groups.Signals.Name = 'In_Value_Wiper'
      | sbobj.Groups.Signals.XData = [0 1 2 3 4 5 6 7 8 9 10 11 12 13 14 15 16 17 18 19 20 21 22 23 24 25]
      | sbobj.Groups.Signals.YData = [1 2 3 4 5 1 2 3 4 5 1 2 3 4 5 1 2 3 4 5 1 2 3 4 5 2]
      | sbobj.Groups.TimeRange = [0 25]
  In_Value_Wiper : Outport  Tag=STV Outport
  wires:
  FromWs/1 -> Demux/1
  Demux/1 -> In_Value_Wiper/1

== system Automated_BCM_Integrated_2020b/BCM_IN_Ports/Signal Builder ==
  Demux : Demux  Tag=STV Demux  Outputs=2
      settings: DisplayOption=none
  FromWs : FromWorkspace  Tag=STV FromWs  VariableName=tuvar
      SigBuilderData=|
      | common.afterFinalStr = 'Extrapolate'
      | common.sampleTime = 0
      | dataSet.timeRange = [0 10]
      | dataSet.name = 'Group 1'
      | sbobj.Groups.Name = 'Group 1'
      | sbobj.Groups.Signals(1).Name = 'In_Su_Roof1'
      | sbobj.Groups.Signals(1).XData = [0 1 2 3 4 5 6 7 8 9 10 11 12 13 14 15 16 17 18 19 20 21 22 23 24 25 26 27 28 29 30 31 32 33 34 35 36 37 38 39 40 41 42 43 44 45]
      | sbobj.Groups.Signals(1).YData = [0 1 2 3 3 2 1 1 0 1 2 3 3 2 1 0 1 1 2 3 3 2 1 0 1 2 3 3 2 2 1 1 0 0 1 1 2 2 3 3 2 2 1 1 1 0]
      | sbobj.Groups.Signals(2).Name = 'I_Sensor1'
      | sbobj.Groups.Signals(2).XData = [0 1 2 3 4 5 6 7 8 9 10 11 12 13 14 15 16 17 18 19 20 21 22 23 24 25 26 27 28 29 30 31 32 33 34 35 36 37 38 39 40 41 42 43 44 45]
      | sbobj.Groups.Signals(2).YData = [0 0 0 0 0 0 0 1 1 1 1 0 0 0 0 0 1 1 0 0 0 1 1 0 0 0 0 0 1 1 0 0 0 0 1 1 1 0 0 0 0 0 1 1 1 0]
      | sbobj.Groups.TimeRange = [0 45]
  In_Su_Roof1 : Outport  Tag=STV Outport
  I_Sensor1 : Outport  Tag=STV Outport  Port=2
  wires:
  FromWs/1 -> Demux/1
  Demux/1 -> In_Su_Roof1/1
  Demux/2 -> I_Sensor1/1

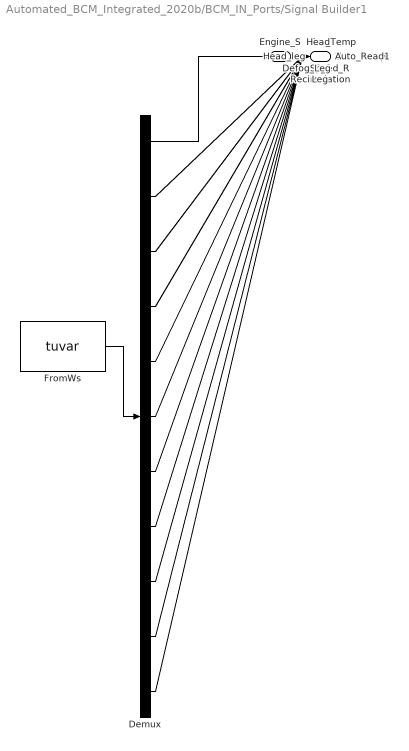
== system Automated_BCM_Integrated_2020b/BCM_IN_Ports/Signal Builder1 ==
  Demux : Demux  Tag=STV Demux  Outputs=11
      settings: DisplayOption=none
  FromWs : FromWorkspace  Tag=STV FromWs  VariableName=tuvar
      SigBuilderData=|
      | common.afterFinalStr = 'Extrapolate'
      | common.sampleTime = 0
      | dataSet.timeRange = [0 36]
      | dataSet.name = 'Group 1'
      | sbobj.Groups.Name = 'Group 1'
      | sbobj.Groups.Signals(1).Name = '      Engine_S  '
      | sbobj.Groups.Signals(1).XData = [0 2 4 6 8 10 12 14 16 18 20 22 24 26 28 30 32 34 36 38 40 42 44 46 48 50 52 54 56 58 60 62 64 66 68 70 72 73 74 75 76 77 78 79 80]
      | sbobj.Groups.Signals(1).YData = [1 1 0 0 0 0 0 0 0 0 0 1 1 1 1 1 1 1 1 1 1 1 1 1 1 1 1 1 1 1 1 1 1 1 1 1 1 1 0 0 1 1 0 1 0]
      | sbobj.Groups.Signals(2).Name = 'AC_S'
      | sbobj.Groups.Signals(2).XData = [0 4 6 8 10 12 14 16 18 20 22 24 26 28 30 32 34 36 38 40 42 44 46 48 50 52 54 56 58 60 62 64 66 68 70 72 73 74 75 76 77 78 79 80]
      | sbobj.Groups.Signals(2).YData = [1 1 0 1 0 1 0 1 0 1 0 0 0 0 0 0 0 0 0 0 1 1 1 1 1 1 1 1 1 1 1 1 0 1 1 1 1 0 1 1 1 1 1 0]
      | sbobj.Groups.Signals(3).Name = 'Car_Temp'
      | sbobj.Groups.Signals(3).XData = [0 2 4 6 8 10 12 14 16 18 20 22 24 26 28 30 32 34 36 38 40 42 44 46 48 50 52 54 56 58 60 62 64 66 68 70 72 73 74 75 76 77 78 79 80]
      | sbobj.Groups.Signals(3).YData = [25 25 0 24 32 50 29 0 25 26 32 25 40 24 31 25 35 24 26 24 29 32 40 28 31 42 28 31 42 -40 20 40 25 14 25 15 50 50 49 25 25 42 45 15 15]
      | sbobj.Groups.Signals(4).Name = 'User_Temp'
      | sbobj.Groups.Signals(4).XData = [0 2 4 6 8 10 12 14 16 18 20 22 24 26 28 30 32 34 36 38 40 42 44 46 48 50 52 54 56 58 60 62 64 66 68 70 72 73 74 75 76 77 78 79 80]
      | sbobj.Groups.Signals(4).YData = [22 22 0 24 34 0 32 50 25 28 25 22 18 24 30 18 29 26 30 28 24 34 21 29 32 26 29 20 26 28 45 25 24 72 39 25 25 40 45 0 45 1000 255 25 54]
      | sbobj.Groups.Signals(5).Name = 'Recirculation'
      | sbobj.Groups.Signals(5).XData = [0 2 4 6 8 10 12 14 16 18 20 22 24 26 28 30 32 34 36 38 40 42 44 46 48 50 52 54 56 58 60 62 64 66 68 70 72 73 74 75 76 77 78 79 80]
      | sbobj.Groups.Signals(5).YData = [1 1 0 0 1 1 0 1 0 1 0 1 0 0 1 0 1 0 0 1 0 0 0 0 1 0 0 0 0 0 0 1 0 1 0 0 0 1 0 1 1 1 1 0 45584]
      | sbobj.Groups.Signals(6).Name = 'Speed_R'
      | sbobj.Groups.Signals(6).XData = [0 2 4 6 8 10 12 14 16 18 20 22 24 26 28 30 32 34 36 38 40 42 44 46 48 50 52 54 56 58 60 62 64 66 68 70 72 73 74 75 76 77 78 79 80]
      | sbobj.Groups.Signals(6).YData = [0 0 1 0 2 1 0 0 1 0 2 3 0 2 0 2 0 3 0 0 3 0 0 2 0 2 0 3 2 3 2 4 5 0 2 1 2 0 0 0 0 0 0 7 165]
      | sbobj.Groups.Signals(7).Name = 'Head'
      | sbobj.Groups.Signals(7).XData = [0 4 6 8 10 12 14 16 18 20 22 24 26 28 30 32 34 36 38 40 42 44 46 48 50 52 54 56 58 60 62 64 66 68 70 72 73 74 75 76 77 78 79 80]
      | sbobj.Groups.Signals(7).YData = [1 1 0 1 0 0 0 1 0 1 0 1 0 1 0 1 0 0 0 0 1 0 1 1 0 0 0 0 0 0 0 2 0 1 0 0 1 0 0 0 0 0 4 55]
      | sbobj.Groups.Signals(8).Name = 'Head_leg'
      | sbobj.Groups.Signals(8).XData = [0 2 4 6 8 10 12 14 16 18 20 22 24 26 28 30 32 34 36 38 40 42 44 46 48 50 52 54 56 58 60 62 64 66 68 70 72 73 74 75 76 77 78 79 80]
      | sbobj.Groups.Signals(8).YData = [0 0 1 0 0 0 0 1 0 0 0 0 0 0 0 0 0 1 0 0 0 0 0 0 0 1 0 1 0 0 0 0 0 0 0 0 1 0 0 0 3 0 0 0 0]
      | sbobj.Groups.Signals(9).Name = 'Leg'
      | sbobj.Groups.Signals(9).XData = [0 4 6 8 10 12 14 16 18 20 22 24 26 28 30 32 34 36 38 40 42 44 46 48 50 52 54 56 58 60 62 64 66 68 70 72 73 74 75 76 77 78 79 80]
      | sbobj.Groups.Signals(9).YData = [0 0 1 0 1 0 0 1 0 0 0 0 0 0 1 0 0 1 0 0 0 1 0 0 0 0 0 1 0 0 1 0 0 1 0 0 0 0 0 1 0 0 0 0]
      | sbobj.Groups.Signals(10).Name = 'Defog_Leg'
      | sbobj.Groups.Signals(10).XData = [0 2 4 6 8 10 12 14 16 18 20 22 24 26 28 30 32 34 36 38 40 42 44 46 48 50 52 54 56 58 60 62 64 66 68 70 72 73 74 75 76 77 78 79 80]
      | sbobj.Groups.Signals(10).YData = [0 0 1 0 1 0 0 0 0 1 0 0 0 0 0 0 0 0 0 1 0 0 0 1 0 0 0 0 0 1 0 0 0 0 1 0 0 0 0 1 0 0 0 0 0]
      | sbobj.Groups.Signals(11).Name = 'Auto_Read1'
      | sbobj.Groups.Signals(11).XData = [0 4 6 8 10 12 14 16 18 20 22 24 26 28 30 32 34 36 38 40 42 44 46 48 50 52 54 56 58 60 62 64 66 68 70 72 73 74 75 76 77 78 79 80]
      | sbobj.Groups.Signals(11).YData = [0 0 0 0 0 1 0 0 0 1 0 0 0 0 0 0 0 0 0 1 0 0 0 0 0 0 0 0 0 1 0 1 0 1 1 0 0 1 0 0 4 0 0 0]
      | sbobj.Groups.TimeRange = [0 36]
  "      Engine_S  " : Outport  Tag=STV Outport
  AC_S : Outport  Tag=STV Outport  Port=2
  Car_Temp : Outport  Tag=STV Outport  Port=3
  User_Temp : Outport  Tag=STV Outport  Port=4
  Recirculation : Outport  Tag=STV Outport  Port=5
  Speed_R : Outport  Tag=STV Outport  Port=6
  Head : Outport  Tag=STV Outport  Port=7
  Head_leg : Outport  Tag=STV Outport  Port=8
  Leg : Outport  Tag=STV Outport  Port=9
  Defog_Leg : Outport  Tag=STV Outport  Port=10
  Auto_Read1 : Outport  Tag=STV Outport  Port=11
  wires:
  FromWs/1 -> Demux/1
  Demux/1 -> "      Engine_S  "/1
  Demux/2 -> AC_S/1
  Demux/3 -> Car_Temp/1
  Demux/4 -> User_Temp/1
  Demux/5 -> Recirculation/1
  Demux/6 -> Speed_R/1
  Demux/7 -> Head/1
  Demux/8 -> Head_leg/1
  Demux/9 -> Leg/1
  Demux/10 -> Defog_Leg/1
  Demux/11 -> Auto_Read1/1

== system Automated_BCM_Integrated_2020b/BCM_IN_Ports/Square_Signals ==
  Demux : Demux  Tag=STV Demux  Outputs=3
      settings: DisplayOption=none
  FromWs : FromWorkspace  Tag=STV FromWs  VariableName=tuvar
      SigBuilderData=|
      | common.afterFinalStr = 'Extrapolate'
      | common.sampleTime = 0
      | dataSet.timeRange = [0 100]
      | dataSet.name = 'Sheet1'
      | sbobj.Name = 'Signal Builder'
      | sbobj.Groups.Name = 'Sheet1'
      | sbobj.Groups.Signals(1).Name = 'Vehicle_Speed'
      | sbobj.Groups.Signals(1).XData = [0 5 10 15 20 25 30 35 40 45 50 55 60 65 70 75 80 85 90 95 100]
      | sbobj.Groups.Signals(1).YData = [0 37 37 50 50 50 50 50 50 50 50 50 50 50 50 50 50 50 50 50 50]
      | sbobj.Groups.Signals(2).Name = 'Cruise_Control'
      | sbobj.Groups.Signals(2).XData = [0 5 5 10 10 15 15 20 20 25 25 30 35 40 45 50 50 55 60 65 70 75 80 85 90 95 100]
      | sbobj.Groups.Signals(2).YData = [0 0 1 1 0 0 1 1 0 0 1 1 1 1 1 1 0 0 0 0 0 0 0 0 0 0 0]
      | sbobj.Groups.Signals(3).Name = 'Set_Res_Control'
      | sbobj.Groups.Signals(3).XData = [0 5 10 15 15 20 20 25 30 35 40 45 50 55 60 60 65 65 70 75 80 85 90 95 100]
      | sbobj.Groups.Signals(3).YData = [0 0 0 0 1 1 0 0 0 0 0 0 0 0 0 1 1 0 0 0 0 0 0 0 0]
      | sbobj.Groups.TimeRange = [0 100]
  Vehicle_Speed : Outport  Tag=STV Outport
  Cruise_Control : Outport  Tag=STV Outport  Port=2
  Set_Res_Control : Outport  Tag=STV Outport  Port=3
  wires:
  FromWs/1 -> Demux/1
  Demux/1 -> Vehicle_Speed/1
  Demux/2 -> Cruise_Control/1
  Demux/3 -> Set_Res_Control/1

== system Automated_BCM_Integrated_2020b/BCM_Controller_and_Plant/BCM_Cruise_Control/If Action Subsystem ==
  In1 : Inport
  Action Port : ActionPort  ActionPortLabel=if(u1 == 1)
  Out1 : Outport
  wires:
  In1/1 -> Out1/1

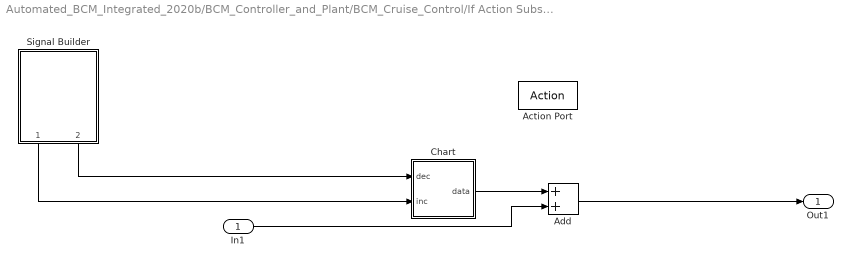
== system Automated_BCM_Integrated_2020b/BCM_Controller_and_Plant/BCM_Cruise_Control/If Action Subsystem1 ==
  In1 : Inport
  Action Port : ActionPort  ActionPortLabel=if(u1 == 1)
  Add : Sum
  Chart : Stateflow chart  TreatAsAtomicUnit=on
  Signal Builder : Subsystem  Tag=STV Subsys  LoadFcn=sigbuilder_block('load');  StartFcn=sigbuilder_block('start');  StopFcn=sigbuilder_block('stop');  ClipboardFcn=sigbuilder_block('clipboard');  mask(Sigbuilder block){tuvar=[0:10]}
      mask help: Simulink:masks:SigbuilderBlock_MD
      mask init:
      | if ~strcmp(get_param(bdroot(gcbh),'SimulationStatus'),'stopped') tuvar = sigbuilder_block('maskInit'); end
      settings: CopyFcn=sigbuilder_block('copy');  DeleteFcn=sigbuilder_block('delete');  ModelCloseFcn=sigbuilder_block('modelClose');  PreSaveFcn=sigbuilder_block('preSave');  PauseFcn=sigbuilder_block('pause');  ContinueFcn=sigbuilder_block('continue');  NameChangeFcn=sigbuilder_block('namechange');  OpenFcn=sigbuilder_block('open',[6 30 1428 681.75 ]);  CloseFcn=sigbuilder_block('close');
      mask Display: plot(0, 0, 100, 100,[2, 2, 32, 32, 2], [68, 8, 8, 68, 68],[32, 2], [38, 38], [32, 19, 2],[53, 60, 44], [32, 17, 17, 2],[16, 16, 31, 31]);txt = getActiveGroup(gcbh);text(2, 100, txt,'verticalAlignment', 'top');
  Out1 : Outport
  wires:
  Signal Builder/1(Plus_Or_Resume) -> Chart/2(inc)
  Add/1 -> Out1/1
  Signal Builder/2(Set_Or_Minus) -> Chart/1(dec)
  Chart/1(data) -> Add/1
  In1/1 -> Add/2

== system Automated_BCM_Integrated_2020b/BCM_Controller_and_Plant/BCM_HO_Controller/BCM_HO_BABU ==
  In1 : Inport
  Out1 : Outport
  wires:
  In1/1 -> Out1/1

== system Automated_BCM_Integrated_2020b/BCM_Controller_and_Plant/BCM_HO_Controller/BCM_HO_DRBU ==
  In1 : Inport
  Out1 : Outport
  wires:
  In1/1 -> Out1/1

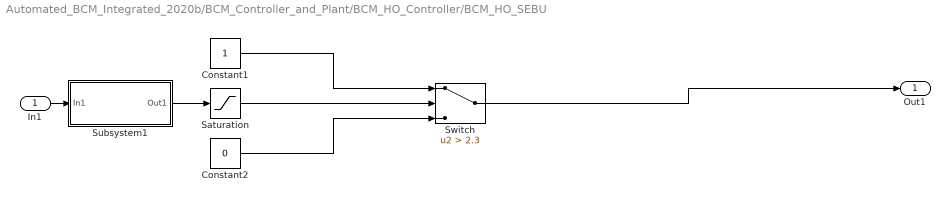
== system Automated_BCM_Integrated_2020b/BCM_Controller_and_Plant/BCM_HO_Controller/BCM_HO_SEBU ==
  In1 : Inport
  Constant1 : Constant
  Constant2 : Constant  Value=0
  Saturation : Saturate  UpperLimit=3.6  LowerLimit=0
  Subsystem1 : Subsystem
  Switch : Switch  Criteria=u2 > Threshold  Threshold=2.3
  Out1 : Outport
  wires:
  In1/1 -> Subsystem1/1(In1)
  Saturation/1 -> Switch/2
  Constant1/1 -> Switch/1
  Constant2/1 -> Switch/3
  Switch/1 -> Out1/1
  Subsystem1/1(Out1) -> Saturation/1

== system Automated_BCM_Integrated_2020b/BCM_Controller_and_Plant/BCM_HO_Controller/BCM_HO_STBU ==
  In1 : Inport
  Out1 : Outport
  wires:
  In1/1 -> Out1/1

== system Automated_BCM_Integrated_2020b/BCM_Controller_and_Plant/BCM_HO_Controller/BCM_HO_out_buttons ==
  In1 : Inport
  Out1 : Outport
  wires:
  In1/1 -> Out1/1

== system Automated_BCM_Integrated_2020b/BCM_Controller_and_Plant/BCM_Cruise_Control/If Action Subsystem1/Signal Builder ==
  Demux : Demux  Tag=STV Demux  Outputs=2
      settings: DisplayOption=none
  FromWs : FromWorkspace  Tag=STV FromWs  VariableName=tuvar
      SigBuilderData=|
      | common.afterFinalStr = 'Extrapolate'
      | common.sampleTime = 0
      | dataSet.timeRange = [0 100]
      | dataSet.name = 'Sheet1'
      | sbobj.Groups.Name = 'Sheet1'
      | sbobj.Groups.Signals(1).Name = 'Plus_Or_Resume'
      | sbobj.Groups.Signals(1).XData = [0 5 10 15 20 25 30 30 35 35 40 45 50 55 60 65 70 75 80 85 90 95 100]
      | sbobj.Groups.Signals(1).YData = [0 0 0 0 0 0 0 1 1 0 0 0 1 0 0 0 0 0 0 0 0 0 0]
      | sbobj.Groups.Signals(2).Name = 'Set_Or_Minus'
      | sbobj.Groups.Signals(2).XData = [0 5 10 15 20 25 30 35 40 40 45 45 50 55 60 65 70 75 80 85 90 95 100]
      | sbobj.Groups.Signals(2).YData = [0 0 0 0 0 0 0 0 0 1 1 0 1 0 0 0 0 0 0 0 0 0 0]
      | sbobj.Groups.TimeRange = [0 100]
  Plus_Or_Resume : Outport  Tag=STV Outport
  Set_Or_Minus : Outport  Tag=STV Outport  Port=2
  wires:
  FromWs/1 -> Demux/1
  Demux/1 -> Plus_Or_Resume/1
  Demux/2 -> Set_Or_Minus/1

== system Automated_BCM_Integrated_2020b/BCM_Controller_and_Plant/BCM_HO_Controller/BCM_HO_SEBU/Subsystem1 ==
  In1 : Inport
  Out1 : Outport
  wires:
  In1/1 -> Out1/1

== stateflow chart Automated_BCM_Integrated_2020b/BCM_Controller_and_Plant/BCM_Cruise_Control/If Action Subsystem1/Chart ==
  state main
    during:
    if inc==1
    data=data+1;
    end
    if dec==1
    data=data-1;
    end
  (default) -> main
  data: dec input; inc input; data output =0

== matlab function Automated_BCM_Integrated_2020b/BCM_Controller_and_Plant/BCM_Sunroof/Function_Sun ==
  data: u input; y output; v input
function y = fcn(u,v)
if u == 1
    for i = 1:5
        y = u * i;
    end
elseif u == 2
    for i = 1:5
        y = u * i;
    end
elseif u == 3
    for i = 1:5
        y = u * i;
    end
else
    y = u;
end
if v == 1 && u ~= 0
   y = 15;
end

== stateflow chart Automated_BCM_Integrated_2020b/BCM_Controller_and_Plant/Subsystem/AC_control_chart ==
  state Recirculation1
    en:
    Re_Op=0;
  state Recirculation
    en:
    Re_Op = 1;
  state AC_ON
    en:
    blower= 1;
    (default) -> (junction 154) : % blowerSpeed
    (junction 154) -> (junction 155) [order 1] : [Speed_Read==2]
    (junction 154) -> (junction 156) [order 2]
    (junction 155) -> (junction 160) : {Speed_Op=2;}
    (junction 156) -> (junction 157) [order 1] : [Speed_Read==3]
    (junction 156) -> (junction 158) [order 2] : {Speed_Op=1;}
    (junction 157) -> (junction 159) : {Speed_Op=3;}
    (junction 159) -> (junction 158)
    (junction 160) -> (junction 159)
    (junction 158) -> (junction 161)
  state Compressor_cond
    en:
    compressor = 1;
  state HVAC_OFF
    en:
    blower=0;
    compressor=0;
  state Compressor_cond1
    en:
    compressor = 0;
  state Auto_cond
    (default) -> (junction 67) : % Auto_cond
    (junction 67) -> (junction 68) [order 1] : [head == 1 ]
    (junction 67) -> (junction 69) [order 2]
    (junction 68) -> (junction 76) : {Dir_Op = 1;}
    (junction 69) -> (junction 70) [order 1] : [leg == 1]
    (junction 69) -> (junction 71) [order 2]
    (junction 70) -> (junction 75) : {Dir_Op = 2;}
    (junction 71) -> (junction 72) [order 1] : [head_leg == 1]
    (junction 71) -> (junction 73) [order 2]
    (junction 72) -> (junction 74) : {Dir_Op = 3;}
    (junction 73) -> (junction 79) [order 1] : [Defog_leg == 1]
    (junction 73) -> (junction 77) [order 2] : {Dir_Op = 0;}
    (junction 79) -> (junction 78) : {Dir_Op = 4;}
    (junction 78) -> (junction 77)
    (junction 74) -> (junction 78)
    (junction 75) -> (junction 74)
    (junction 76) -> (junction 75)
  Recirculation1 -> AC_ON : after(0.5,usec)
  AC_ON -> Recirculation1 [order 6] : [blower==1&&Re_read==0]
  AC_ON -> Recirculation [order 5] : [blower==1 && Re_read==1]
  Recirculation -> AC_ON : after(0.005,usec)
  AC_ON -> Compressor_cond [order 2] : [User_temp < Sensor_read && compressor ==0 ]
  (default) -> HVAC_OFF
  Compressor_cond -> AC_ON : after(0.005,usec)
  HVAC_OFF -> AC_ON : [Engine == 1 && AC ==1]
  AC_ON -> HVAC_OFF [order 1] : [Engine ==0 || AC == 0]
  AC_ON -> Compressor_cond1 [order 3] : [User_temp >= Sensor_read && compressor ==1]
  Compressor_cond1 -> AC_ON : after(0.005,usec)
  Auto_cond -> AC_ON : after(0.005,usec)
  AC_ON -> Auto_cond [order 4] : [AutoRead==1|| head ==1 || head_leg ==1 || leg == 1 || Defog_leg == 1]
  data: Engine input; AC input; blower output; Sensor_read input; User_temp input; Re_read input; Re_Op output; Speed_Op output; Speed_Read input; compressor output; head input; head_leg input; leg input; Defog_leg input; Dir_Op output; AutoRead input
